simulink model "sl_rrmc2"  (R2015a)
settings: Solver=ode45  StartTime=0.0  StopTime=10.0  RelTol=1e-3
PreLoadFcn:
  | fprintf('*** Loading Puma560 model to workspace\n');
  | mdl_puma560
undefined symbols (not defined in the file): DiscIntNeverNeededParam, p560, qn, transl
libraries: roblocks x5, simulink x1
settings Model: ExtModeTrigMode=oneshot  ExtModeArmWhenConnect=off  Creator=pic  LastModifiedBy=corkep
settings DataIOCC: LimitDataPoints=off  SignalLoggingSaveFormat=ModelDataLogs
settings OptimizationCC: BlockReduction=off  BooleanDataType=off  ExpressionDepthLimit=2147483647  InitFltsAndDblsToZero=on
settings DebuggingCC: SaveWithParameterizedLinksMsg=none  UnderspecifiedInitializationDetection=Classic  MergeDetectMultiDrivingBlocksExec=none  SignalResolutionControl=TryResolveAllWithWarning  MultiTaskDSMMsg=warning  MultiTaskCondExecSysMsg=none  FcnCallInpInsideContextMsg=EnableAllAsWarning  StateNameClashWarn=warning
settings HardwareCC: TargetUnknown=on
settings GRTTargetCC: ModelReferenceCompliant=off  CompOptLevelCompliant=off  CombineOutputUpdateFcns=off  MatFileLogging=off  GRTInterface=on

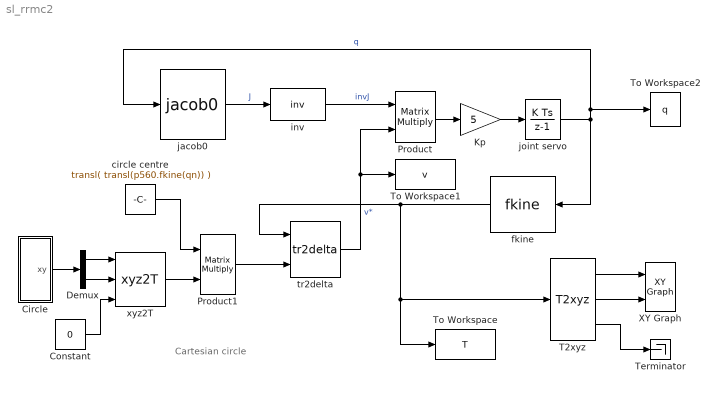
== system sl_rrmc2 ==
  note: Cartesian circle
  Circle : Subsystem  mask{radius=0.05, freq=0.2}
      mask prompts: freq "Frequency (rev/s)"
  Constant : Constant  Value=0
  Demux : Demux  Outputs=2
  Kp : Gain  Gain=5  SaturateOnIntegerOverflow=on  OutDataTypeStr=Inherit: Same as input  ParamDataTypeStr=Inherit: Same as input
  Product : Product  Multiplication=Matrix(*)  SaturateOnIntegerOverflow=on  RndMeth=Zero  InputSameDT=on  OutDataTypeStr=Inherit: Same as first input
  Product1 : Product  Multiplication=Matrix(*)  SaturateOnIntegerOverflow=on  RndMeth=Zero  InputSameDT=on  OutDataTypeStr=Inherit: Same as first input
  T2xyz : roblocks/Toolbox/T2xyz
  Terminator : Terminator
  To Workspace : ToWorkspace  VariableName=T  SampleTime=-1
  To Workspace1 : ToWorkspace  VariableName=v  SampleTime=-1
  To Workspace2 : ToWorkspace  VariableName=q  SampleTime=-1
  XY Graph : simulink/Sinks/XY Graph  xmin=0.5  xmax=0.7  ymin=-0.25  ymax=-0.05  st=-1
  circle centre : Constant  Value=transl( transl(p560.fkine(qn)) )
  fkine : roblocks/Arm/fkine  robot=p560
  inv : MATLABFcn  MATLABFcn=inv  Output1D=off
  "jacob0 " : roblocks/Arm/jacob0   robot=p560
  joint servo : DiscreteIntegrator  InitialCondition=qn'  SampleTime=0.05  ICPrevOutput=DiscIntNeverNeededParam  ICPrevScaledInput=DiscIntNeverNeededParam
  tr2delta : roblocks/Toolbox/tr2delta
  xyz2T : roblocks/Toolbox/xyz2T
  wires:
  joint servo/1 -> To Workspace2/1, "jacob0 "/1, fkine/1  "q"
  T2xyz/1 -> XY Graph/1
  T2xyz/2 -> XY Graph/2
  tr2delta/1 -> Product/2, To Workspace1/1  "v*"
  Demux/1 -> xyz2T/1
  "jacob0 "/1 -> inv/1  "J"
  Product/1 -> Kp/1
  inv/1 -> Product/1  "invJ"
  Kp/1 -> joint servo/1
  Demux/2 -> xyz2T/2
  Circle/1(xy) -> Demux/1
  Constant/1 -> xyz2T/3
  fkine/1 -> tr2delta/1, To Workspace/1, T2xyz/1
  xyz2T/1 -> Product1/2
  circle centre/1 -> Product1/1
  T2xyz/3 -> Terminator/1
  Product1/1 -> tr2delta/2

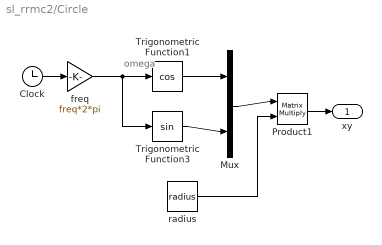
== system sl_rrmc2/Circle ==
  note: omega
  Clock : Clock
  Mux : Mux  Inputs=2
  Product1 : Product  Multiplication=Matrix(*)  RndMeth=Zero
  Trigonometric Function1 : Trigonometry  Operator=cos
  Trigonometric Function3 : Trigonometry
  freq : Gain  Gain=freq*2*pi
  radius : Constant  Value=radius
  xy : Outport
  wires:
  freq/1 -> Trigonometric Function3/1, Trigonometric Function1/1
  Product1/1 -> xy/1
  Clock/1 -> freq/1
  radius/1 -> Product1/2
  Mux/1 -> Product1/1
  Trigonometric Function1/1 -> Mux/1
  Trigonometric Function3/1 -> Mux/2
